simulink model "Phone_A"  (R2023a)
settings: Solver=FixedStepDiscrete  StartTime=0.0  StopTime=inf  RelTol=1e-3
undefined symbols (not defined in the file): DiscIntNeverNeededParam
libraries: androiduilib x5, androidsensorlib x3, androidaudiovideolib x2, androidcommunicationlib x2
settings Model: Creator=mtaru  LastModifiedBy=mtaru
settings OptimizationCC: EnhancedBackFolding=on  PassReuseOutputArgsAs=Individual arguments  ZeroExternalMemoryAtStartup=off  ZeroInternalMemoryAtStartup=off  MaxStackSize=64  OptimizeBlockOrder=speed  DifferentSizesBufferReuse=on  OptimizationCustomize=off  EfficientTunableParamExpr=on
settings DebuggingCC: ParameterTunabilityLossMsg=error
settings HardwareCC: ProdBitPerPointer=32  ProdBitPerSizeT=32  ProdBitPerPtrDiffT=32  ProdLargestAtomicInteger=Long  ProdLargestAtomicFloat=Double  ProdWordSize=32  ProdHWDeviceType=ARM Compatible->ARM Cortex
settings SFSimCC: MATLABDynamicMemAlloc=off
settings RTWCC: Description=Embedded Coder  SystemTargetFile=ert.tlc  HardwareBoard=Android Device  TLCOptions="-aInlineSetEventsForThisBaseRateFcn=TLC_FALSE -aSuppressMultiTaskScheduler=TLC_FALSE  -aRateBasedStepFcn=0"  TemplateMakefile=ert_default_tmf  RTWVerbose=off  Toolchain=Android SDK/NDK Tools  BuildConfiguration=Faster Runs
settings CodeAppCC: ForceParamTrailComments=on  IgnoreCustomStorageClasses=off  OperatorAnnotations=on  SimulinkDataObjDesc=on  SFDataObjDesc=on  InsertBlockDesc=on
settings ERTTargetCC: SupportVariableSizeSignals=on

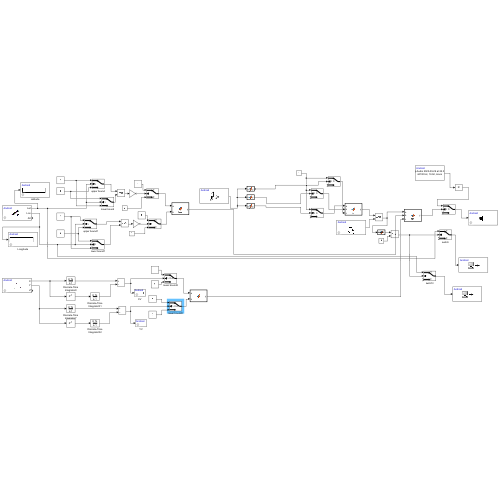
[thumbnail: Simulink's stored preview of the top-level diagram]
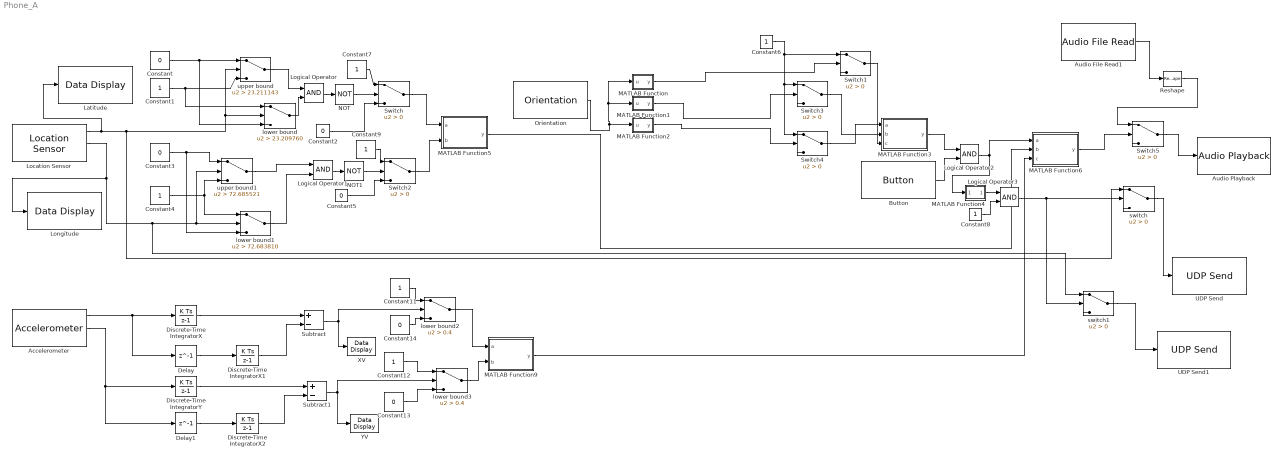
== system Phone_A ==
  Accelerometer : androidsensorlib/Accelerometer  OutputVector=off  SampleTime=0.1  BlockPlatform=Android
  Audio File Read1 : androidaudiovideolib/Audio File Read  FileName=C:\Matlab_Android\WhatsApp Audio 2023-09-29 at 22.37.18.mp3  FrameSize=882
  Audio Playback : androidaudiovideolib/Audio Playback  SampleFreq=44100  AudioSamplingFreq=44100  SampleTime=0.1  DeviceStr=0  QueueDuration=0  BlockPlatform=Android
  Button : androiduilib/Button  ButtonState=Pressed  ButtonId=Phone_A/Button  State=on  SampleTime=0.1  BlockPlatform=Android
  Constant{,2..3,5,13..14} (6 alike) : Constant  Value=0
  Constant{1,4,6..9,11..12} (8 alike) : Constant
  Delay : Delay  DelayLength=1  InitialCondition=0
  Delay1 : Delay  DelayLength=1  InitialCondition=0
  Discrete-Time IntegratorX : DiscreteIntegrator  SampleTime=-1  ICPrevOutput=DiscIntNeverNeededParam  ICPrevScaledInput=DiscIntNeverNeededParam
  Discrete-Time IntegratorX1 : DiscreteIntegrator  SampleTime=-1  ICPrevOutput=DiscIntNeverNeededParam  ICPrevScaledInput=DiscIntNeverNeededParam
  Discrete-Time IntegratorX2 : DiscreteIntegrator  SampleTime=-1  ICPrevOutput=DiscIntNeverNeededParam  ICPrevScaledInput=DiscIntNeverNeededParam
  Discrete-Time IntegratorY : DiscreteIntegrator  SampleTime=-1  ICPrevOutput=DiscIntNeverNeededParam  ICPrevScaledInput=DiscIntNeverNeededParam
  Latitude : androiduilib/Data Display  DataDisplayId=Phone_A/Latitude  Format=Float  Precision=6  SimulateUsing=Code generation  blockPlatform=Android
  Location Sensor : androidsensorlib/Location Sensor  OutputVector=off  SampleTime=0.01  BlockPlatform=Android
  Logical Operator{,1..3} (4 alike) : Logic  AllPortsSameDT=off  OutDataTypeStr=boolean
  Longitude : androiduilib/Data Display  DataDisplayId=Phone_A/Longitude  Format=Float  Precision=6  SimulateUsing=Code generation  blockPlatform=Android
  MATLAB Function : MATLAB Function  TreatAsAtomicUnit=on
  MATLAB Function1 : MATLAB Function  TreatAsAtomicUnit=on
  MATLAB Function2 : MATLAB Function  TreatAsAtomicUnit=on
  MATLAB Function3 : MATLAB Function  TreatAsAtomicUnit=on
  MATLAB Function4 : MATLAB Function  TreatAsAtomicUnit=on
  MATLAB Function5 : MATLAB Function  TreatAsAtomicUnit=on
  MATLAB Function6 : MATLAB Function  TreatAsAtomicUnit=on
  MATLAB Function9 : MATLAB Function  TreatAsAtomicUnit=on
  NOT : Logic  Operator=NOT  IconShape=distinctive  AllPortsSameDT=off  OutDataTypeStr=boolean
  NOT1 : Logic  Operator=NOT  IconShape=distinctive  AllPortsSameDT=off  OutDataTypeStr=boolean
  Orientation : androidsensorlib/Orientation  SampleTime=0.1
  Reshape : Reshape  OutputDimensionality=Customize  OutputDimensions=[441,2]
  Subtract : Sum  Inputs=+-
  Subtract1 : Sum  Inputs=+-
  Switch{,1..5} (6 alike) : Switch  Criteria=u2 > Threshold  SaturateOnIntegerOverflow=off  InputSameDT=off
  UDP Send : androidcommunicationlib/UDP Send  remoteURL='10.7.4.116'  remotePort=25000  localURL='0.0.0.0'  localPortSource=Automatically determine  localPort=-1  sampletime=-1  blockPlatform=Android  separateLengthPort=0
  UDP Send1 : androidcommunicationlib/UDP Send  remoteURL='10.7.4.116'  remotePort=25001  localURL='0.0.0.0'  localPortSource=Automatically determine  localPort=-1  sampletime=-1  blockPlatform=Android  separateLengthPort=0
  XV : androiduilib/Data Display  DataDisplayId=Phone_A/XV  Format=Float  Precision=6  SimulateUsing=Code generation  blockPlatform=Android
  YV : androiduilib/Data Display  DataDisplayId=Phone_A/YV  Format=Float  Precision=6  SimulateUsing=Code generation  blockPlatform=Android
  lower bound : Switch  Criteria=u2 > Threshold  Threshold=23.209760  SaturateOnIntegerOverflow=off  InputSameDT=off
  lower bound1 : Switch  Criteria=u2 > Threshold  Threshold=72.683810  SaturateOnIntegerOverflow=off  InputSameDT=off
  lower bound2 : Switch  Criteria=u2 > Threshold  Threshold=0.4  SaturateOnIntegerOverflow=off  InputSameDT=off
  lower bound3 : Switch  Criteria=u2 > Threshold  Threshold=0.4  SaturateOnIntegerOverflow=off  InputSameDT=off
  switch : Switch  Criteria=u2 > Threshold  SaturateOnIntegerOverflow=off  InputSameDT=off
  switch1 : Switch  Criteria=u2 > Threshold  SaturateOnIntegerOverflow=off  InputSameDT=off
  upper bound : Switch  Criteria=u2 > Threshold  Threshold=23.211143  SaturateOnIntegerOverflow=off  InputSameDT=off
  upper bound1 : Switch  Criteria=u2 > Threshold  Threshold=72.685521  SaturateOnIntegerOverflow=off  InputSameDT=off
  wires:
  Location Sensor/1 -> Latitude/1, switch/1, lower bound/2, upper bound/2
  Constant/1 -> lower bound/3, upper bound/1
  Constant1/1 -> upper bound/3, lower bound/1
  upper bound/1 -> Logical Operator/1
  lower bound/1 -> Logical Operator/2
  Logical Operator/1 -> NOT/1
  NOT/1 -> Switch/2
  Constant2/1 -> Switch/3
  Constant5/1 -> Switch2/3
  lower bound1/1 -> Logical Operator1/2
  Constant3/1 -> upper bound1/1, lower bound1/3
  NOT1/1 -> Switch2/2
  Logical Operator1/1 -> NOT1/1
  Constant4/1 -> lower bound1/1, upper bound1/3
  upper bound1/1 -> Logical Operator1/1
  Location Sensor/2 -> Longitude/1, switch1/1, lower bound1/2, upper bound1/2
  MATLAB Function1/1(y) -> Switch3/2
  Orientation/1 -> MATLAB Function2/1(u), MATLAB Function/1(u), MATLAB Function1/1(u)
  MATLAB Function/1(y) -> Switch1/2
  Discrete-Time IntegratorX/1 -> Subtract/1
  Subtract/1 -> lower bound2/2, XV/1
  Discrete-Time IntegratorY/1 -> Subtract1/1
  Subtract1/1 -> lower bound3/2, YV/1
  Accelerometer/2 -> Delay1/1, Discrete-Time IntegratorY/1
  Accelerometer/1 -> Delay/1, Discrete-Time IntegratorX/1
  MATLAB Function2/1(y) -> Switch4/2
  Constant6/1 -> Switch1/1, Switch4/1, Switch3/1
  Switch4/1 -> MATLAB Function3/1(a)
  Switch3/1 -> MATLAB Function3/2(b)
  Switch1/1 -> MATLAB Function3/3(c)
  Switch5/1 -> Audio Playback/1
  Audio File Read1/1 -> Reshape/1
  Reshape/1 -> Switch5/1
  MATLAB Function3/1(y) -> Logical Operator2/1
  Button/1 -> Logical Operator2/2
  Logical Operator2/1 -> MATLAB Function4/1(input), MATLAB Function6/1(a)
  MATLAB Function4/1(output) -> Logical Operator3/1
  Constant8/1 -> Logical Operator3/2
  Switch/1 -> MATLAB Function5/1(a)
  Switch2/1 -> MATLAB Function5/2(b)
  Constant9/1 -> Switch2/1
  Constant7/1 -> Switch/1
  MATLAB Function6/1(y) -> Switch5/2
  Delay/1 -> Discrete-Time IntegratorX1/1
  Discrete-Time IntegratorX1/1 -> Subtract/2
  Delay1/1 -> Discrete-Time IntegratorX2/1
  Discrete-Time IntegratorX2/1 -> Subtract1/2
  switch/1 -> UDP Send/1
  Constant12/1 -> lower bound3/1
  Constant11/1 -> lower bound2/1
  Constant13/1 -> lower bound3/3
  Constant14/1 -> lower bound2/3
  lower bound2/1 -> MATLAB Function9/1(a)
  lower bound3/1 -> MATLAB Function9/2(b)
  MATLAB Function9/1(y) -> MATLAB Function6/3(c)
  MATLAB Function5/1(y) -> MATLAB Function6/2(b)
  Logical Operator3/1 -> switch1/2, switch/2
  switch1/1 -> UDP Send1/1

== matlab function Phone_A/MATLAB Function1 ==
  data: u input; y output
function y = fcn(u)
    x = u(2);
    if abs(x) > 40
        y = 1;
    else
        y = 0;
    end
end

== matlab function Phone_A/MATLAB Function ==
  data: u input; y output
function y = fcn(u)
    x = u(1);
    if abs(x) > 40
        y = 1;
    else
        y = 0;
    end
end

== matlab function Phone_A/MATLAB Function2 ==
  data: u input; y output
function y = fcn(u)
    x = u(3);
    if abs(x) > 40
        y = 1;
    else
        y = 0;
    end
end

== matlab function Phone_A/MATLAB Function3 ==
  data: a input; b input; c input; y output
function y = fcn(a, b, c)
    
    if (a + b + c > 1)
        y = 1;
    else
        y = 0;
    end
end

== matlab function Phone_A/MATLAB Function4 ==
  data: input input; output output
function output = inputLogic(input)
    % Define a persistent variable to track the time the input has been 1
    persistent time_input_1;

    % If the input is 1, increment the time
    if input == 1
        if isempty(time_input_1)
            time_input_1 = 0;
        else
            time_input_1 = time_input_1 + 0.1; % Assuming a sample time of 0.1 seconds
        end
    else
        time_input_1 = 0; % Reset the time if the input is not 1
    end

    % Check if the input has been 1 for at least 5 seconds
    if time_input_1 >= 5
        output = 1;
    else
        output = 0;
    end
end

== matlab function Phone_A/MATLAB Function5 ==
  data: a input; b input; y output
function y = fcn(a, b)
    
    if (a + b >= 1)
        y = 1;
    else
        y = 0;
    end
end

== matlab function Phone_A/MATLAB Function6 ==
  data: a input; b input; c input; y output
function y = fcn(a, b , c)
    
    if (a + b + c  >=1)
        y = 1;
    else
        y = 0;
    end
end

== matlab function Phone_A/MATLAB Function9 ==
  data: a input; b input; y output
function y = fcn(a, b)
    
    if (a + b >= 1)
        y = 1;
    else
        y = 0;
    end
end
